simulink model "EarlyReturn16_2018a"  (R2018a)
settings: Solver=VariableStepAuto  StartTime=0.0  StopTime=0.1  RelTol=1e-3
settings Model: Creator=BEAR  LastModifiedBy=bzhan

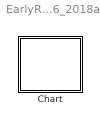
== system EarlyReturn16_2018a ==
  Chart : Stateflow chart  TreatAsAtomicUnit=on

== stateflow chart EarlyReturn16_2018a/Chart ==
  state A
    en: f("en_A")
    ex: f("ex_A")
    state A1
      en: f("en_A1")
      ex: f("ex_A1")
    state A4
      en: f("en_A4")
      ex: f("ex_A4")
    state A3
      en: f("en_A3")
    state A2
      en: f("en_A2")
      ex: f("ex_A2")
    (default) -> A1 : {x=1;}
    A1 -> A2 [order 3]
    A1 -> (junction 12) [order 2] : [x>0]{f("outA1")}
    A1 -> A3 [order 1] : E[x>0]
    (junction 12) -> A4 : {E;f("E")}
    A2 -> (junction 12) [order 2] : [x<0]{f("outA2")}
    A2 -> A3 [order 1] : E[x<0]
  (default) -> A
  data: s function_input; x local
  events: E local FUNCTION_CALL_EVENT
  function f(s):
    | function f(s)
    |   fprintf(s+"\n");
